simulink subsystem "RT_forces_moments"  (R2025a)
settings: Solver=VariableStepAuto  StartTime=0.0  StopTime=10.0  RelTol=1e-3
undefined symbols (not defined in the file): RT_vectorHub2CG, T_Hub2Body
settings Model: DataDictionary=MainRotor.sldd  EnableAccessToBaseWorkspace=off  DefaultTestHarness=MR_forces_moments_Harness1  Creator=tunglt60  LastModifiedBy=tunglt60

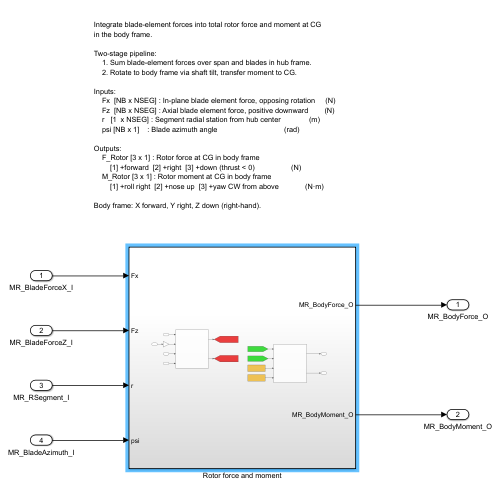
[thumbnail: Simulink's stored preview of the top-level diagram]
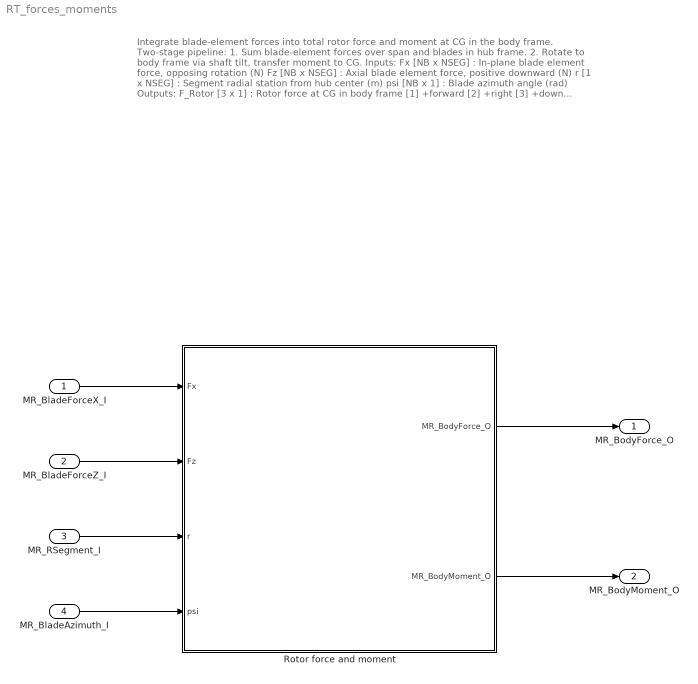
== system RT_forces_moments ==
  note: Integrate blade-element forces into total rotor force and moment at CG
      | in the body frame.
      |
      | Two-stage pipeline:
      | 1. Sum blade-element forces over span and blades in hub frame.
      | 2. Rotate to body frame via shaft tilt, transfer moment to CG.
      |
      | Inputs:
      | Fx [NB x NSEG] : In-plane blade element force, opposing rotation (N)
      | Fz [NB x NSEG] : Axial blade element force, positive downward (N)
      | r [1 x NSEG] : Segment radial station from hub center (m)
      | psi [NB x 1] : Blade azimuth angle (rad)
      |
      | Outputs:
      | F_Rotor [3 x 1] : Rotor force at CG in body frame
      | [1] +forward [2] +right [3] +down (thrust < 0) (N)
      | M_Rotor [3 x 1] : Rotor moment at CG in body frame
      | [1] +roll right [2] +nose up [3] +yaw CW from above (N·m)
      |
      | Body frame: X forward, Y right, Z down (right-hand).
  MR_BladeForceX_I : Inport
  MR_BladeForceZ_I : Inport  Port=2
  MR_RSegment_I : Inport  Port=3
  MR_BladeAzimuth_I : Inport  Port=4
  Rotor force and moment : Subsystem
  MR_BodyForce_O : Outport
  MR_BodyMoment_O : Outport  Port=2
  wires:
  Rotor force and moment/2(MR_BodyMoment_O) -> MR_BodyMoment_O/1
  Rotor force and moment/1(MR_BodyForce_O) -> MR_BodyForce_O/1
  MR_RSegment_I/1 -> Rotor force and moment/3(r)
  MR_BladeForceX_I/1 -> Rotor force and moment/1(Fx)
  MR_BladeForceZ_I/1 -> Rotor force and moment/2(Fz)
  MR_BladeAzimuth_I/1 -> Rotor force and moment/4(psi)

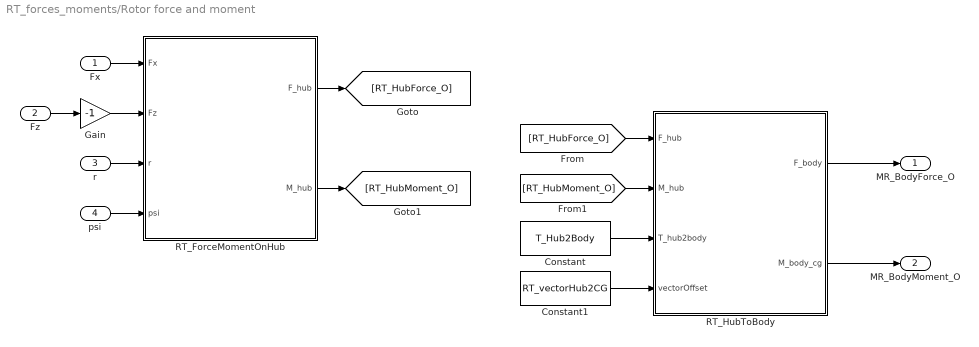
== system RT_forces_moments/Rotor force and moment ==
  Fx : Inport
  Fz : Inport  Port=2
  r : Inport  Port=3
  psi : Inport  Port=4
  Constant : Constant  Value=T_Hub2Body
  Constant1 : Constant  Value=RT_vectorHub2CG
  Gain : Gain  Gain=-1
  RT_ForceMomentOnHub : MATLAB Function  TreatAsAtomicUnit=on
  RT_HubToBody : MATLAB Function  TreatAsAtomicUnit=on
  MR_BodyForce_O : Outport
  MR_BodyMoment_O : Outport  Port=2
  wires:
  RT_HubToBody/1(F_body) -> MR_BodyForce_O/1
  RT_HubToBody/2(M_body_cg) -> MR_BodyMoment_O/1
  [RT_HubMoment_O] -> RT_HubToBody/2(M_hub)
  RT_ForceMomentOnHub/2(M_hub) -> [RT_HubMoment_O]
  [RT_HubForce_O] -> RT_HubToBody/1(F_hub)
  RT_ForceMomentOnHub/1(F_hub) -> [RT_HubForce_O]
  psi/1 -> RT_ForceMomentOnHub/4(psi)
  r/1 -> RT_ForceMomentOnHub/3(r)
  Fz/1 -> Gain/1
  Fx/1 -> RT_ForceMomentOnHub/1(Fx)
  Constant/1 -> RT_HubToBody/3(T_hub2body)
  Constant1/1 -> RT_HubToBody/4(vectorOffset)
  Gain/1 -> RT_ForceMomentOnHub/2(Fz)

== matlab function RT_forces_moments/Rotor force and moment/RT_HubToBody ==
  data: F_hub input; M_hub input; T_hub2body input; vectorOffset input; F_body output; M_body_cg output
function [F_body, M_body_cg] = RT_HubToBody(F_hub, M_hub, T_hub2body, vectorOffset)
%MR_HUBTOBODY Transform rotor forces and moments from hub frame to body frame at CG.
%
%   [F_body, M_body_cg] = MR_HubToBody(F_hub, M_hub, shaft_tilt, r_hub)
%   performs two operations:
%       1. Rotate hub-frame vectors into body frame (shaft tilt).
%       2. Transfer moments from hub location to CG (moment arm offset).
%
%   Inputs:
%       F_hub      - [3 x 1] Rotor force in hub frame                 (N)
%                      from MR_ForceMomentOnHub
%       M_hub      - [3 x 1] Rotor moment in hub frame                (N·m)
%                      from MR_ForceMomentOnHub
%       shaft_tilt - [1 x 1] Forward shaft tilt angle, positive       (rad)
%                      forward (shaft top tilts toward nose)
%       r_hub      - [3 x 1] Position vector FROM CG TO hub           (m)
%                      expressed in body frame [Xh; Yh; Zh]
%                      Xh > 0 : hub is forward of CG
%                      Yh > 0 : hub is right of CG
%                      Zh < 0 : hub is above CG (typical)
%
%   Outputs:
%       F_body     - [3 x 1] Total rotor force in body frame          (N)
%           [1] Fx : forward  (+forward)
%           [2] Fy : lateral  (+right)
%           [3] Fz : axial    (+down, thrust is negative)
%
%       M_body_cg  - [3 x 1] Total rotor moment at CG in body frame   (N·m)
%           [1] Mx : roll   (+roll right)
%           [2] My : pitch  (+nose down)
%           [3] Mz : yaw    (+yaw CW from above)
%
%   See also: MR_ForceMomentOnHub

% -------------------------------------------------------------------------
%   Author  : [TungLT60]
%   Created : 2026-04-16
% -------------------------------------------------------------------------

    %% Input validation
    assert(isequal(size(F_hub), [3, 1]), ...
        'MR_HubToBody:dimMismatch', 'F_hub must be [3 x 1].');
    assert(isequal(size(M_hub), [3, 1]), ...
        'MR_HubToBody:dimMismatch', 'M_hub must be [3 x 1].');
    assert(isscalar(shaft_tilt_deg), ...
        'MR_HubToBody:dimMismatch', 'shaft_tilt must be scalar.');
    assert(isequal(size(r_hub), [3, 1]), ...
        'MR_HubToBody:dimMismatch', 'r_hub must be [3 x 1].');

    %% Step 2 — Rotate hub-frame vectors into body frame
    F_body       = T_hub2body * F_hub;
    M_hub_inbody = T_hub2body * M_hub;

    %% Step 3 — Transfer moment from hub to CG
    %   M_cg = M_hub + r_hub × F_body
    %
    %   Skew-symmetric matrix [r×] such that [r×]·v = r × v :
    %
    %          [  0   -rz   ry ]
    %   [r×] = [  rz   0   -rx ]
    %          [ -ry   rx   0  ]

    rx = vectorOffset(1);
    ry = vectorOffset(2);
    rz = vectorOffset(3);

    r_cross = [  0   -rz   ry ;
                rz    0   -rx ;
               -ry   rx    0  ];

    M_body_cg = M_hub_inbody + r_cross * F_body;

end

== matlab function RT_forces_moments/Rotor force and moment/RT_ForceMomentOnHub ==
  data: Fx input; Fz input; r input; F_hub output; psi input; M_hub output
function [F_hub, M_hub]  = RT_ForceMomentOnHub(Fx, Fz, r, psi)
%MR_FORCEMOMENTONHUB Compute total rotor forces and moments at the hub.
%
%   [F_hub, M_hub] = MR_ForceMomentOnHub(Fx, Fz, r, psi) transforms
%   blade-element aerodynamic forces from the rotating blade frame to the
%   non-rotating hub-fixed frame and sums over all blades.
%
%   Hub-fixed coordinate system (right-hand, NED-like):
%       X_hub : forward   (+nose direction)
%       Y_hub : right     (+starboard)
%       Z_hub : down      (+toward ground)
%
%   Blade-element coordinate system (rotates with blade at azimuth psi):
%       X_elem : in disk plane, perpendicular to blade span, opposing rotation
%       Z_elem : along shaft axis, downward (= Z_hub)
%
%   Inputs:
%       Fx   - [NB x NSEG] In-plane force per element, opposing rotation (N)
%       Fz   - [NB x NSEG] Axial force per element, positive downward    (N)
%       r    - [1  x NSEG] Radial distance from hub center to segment    (m)
%       psi  - [NB x 1]    Azimuth angle of each blade                   (rad)
%
%   Outputs:
%       F_hub - [3 x 1] Total force vector at hub [Fx; Fy; Fz]
%           Fx_hub : forward  force, +forward                           (N)
%           Fy_hub : lateral  force, +right                             (N)
%           Fz_hub : axial    force, +down  (thrust is negative)        (N)
%
%       M_hub - [3 x 1] Total moment vector at hub [Mx; My; Mz]
%           Mx_hub : rolling  moment, +roll right                       (N·m)
%           My_hub : pitching moment, +nose up                          (N·m)
%           Mz_hub : shaft    torque, +yaw CW from above                (N·m)
%                    (typically < 0, since aerodynamic drag opposes rotation)
%
%   Pipiline:
%       1 – Blade-element forces Fx(i,j), Fz(i,j) are given inputs.
%       2 – Integrate along span: sum forces and first moments (force × r).
%       3 – Project each blade's scalars into hub frame via azimuth angle.
%       4 – Sum contributions from all blades.
%
%   Derivation (single element at radial station r, azimuth psi):
%       Position in hub frame : p = r·[cos(psi); sin(psi); 0]
%       X_elem in hub frame   : e = [sin(psi); -cos(psi); 0]
%       Force in hub frame    : F = Fx·e + Fz·[0;0;1]
%       Moment about hub      : M = p × F
%           Mx = +r·Fz·sin(psi)      (flap → roll)
%           My = -r·Fz·cos(psi)      (flap → pitch)
%           Mz = -r·Fx               (drag → torque)
%
%   See also: MR_BladeElementForce <Input from NghiaMB>, MR_HubToBody <next
%   step to calc transfrom from Hub to Body>

% -------------------------------------------------------------------------
%   Author  : [TungLT06]
%   Created : 2026-04-16
% -------------------------------------------------------------------------

    %% 1 - Input validation
    [NB, NSEG] = size(Fx);
    r = r(:)'; % Force r to [1 x NSEG]
    assert(isequal(size(Fz), [NB, NSEG]), ...
        'MR_ForceMomentOnHub:dimMismatch', ...
        'Fz must be [%d x %d], same as Fx.', NB, NSEG);
    assert(isequal(size(r), [1, NSEG]), ...
        'MR_ForceMomentOnHub:dimMismatch', ...
        'r must be [1 x %d].', NSEG);
    assert(isequal(size(psi), [NB, 1]), ...
        'MR_ForceMomentOnHub:dimMismatch', ...
        'psi must be [%d x 1].', NB);

    %% 2 – Span integration (per-blade scalars)
    Fx_blade = sum(Fx, 2);           % [NB x 1]  total in-plane force
    Fz_blade = sum(Fz, 2);           % [NB x 1]  total axial force
    Fz_arm = zeros(NB,1);            % [NB x 1]  first moment of axial force   (flap)
    Fx_arm = zeros(NB,1);            % [NB x 1]  first moment of in-plane force (torque)
    for i=1:NB
        Fz_arm(i) = sum(Fz(i,:) .* r,2);              
        Fx_arm(i) = sum(Fx(i,:) .* r,2);             
    end
    %% 3 – Azimuth projection (rotating → hub frame)
    sp = sin(psi);                    % [NB x 1]
    cp = cos(psi);                    % [NB x 1]

    % --- Forces per blade in hub frame ---
    dFx_hub = -Fx_blade .* sp;       % [NB x 1]  X_hub (forward)
    dFy_hub = -Fx_blade .* cp;       % [NB x 1]  Y_hub (right)
    dFz_hub =  Fz_blade;             % [NB x 1]  Z_hub (down)

    % --- Moments per blade about hub ---
    dMx_hub = Fz_arm .* sp;         % [NB x 1]  roll  (flap × sin)
    dMy_hub = Fz_arm .* cp;         % [NB x 1]  pitch (flap × cos)
    dMz_hub = Fx_arm;               % [NB x 1]  torque (drag × arm)

    %% 4 – Sum over all blades
    F_hub = [sum(dFx_hub); ...
             sum(dFy_hub); ...
             sum(dFz_hub)];           % [3 x 1]  (N)

    M_hub = [sum(dMx_hub); ...
             sum(dMy_hub); ...
             sum(dMz_hub)];           % [3 x 1]  (N·m)

end
